simulink model "muxdemux"  (R2019b)
settings: Solver=VariableStepAuto  StartTime=0.0  StopTime=10.0  RelTol=1e-3
settings Model: Creator=Admin  LastModifiedBy=Admin

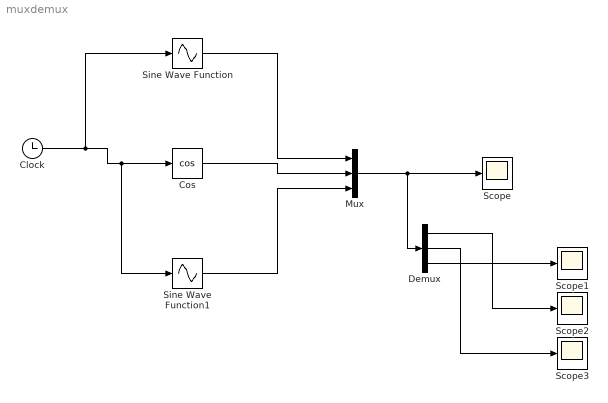
== system muxdemux ==
  Clock : Clock
  Cos : Trigonometry  Operator=cos
  Demux : Demux  Outputs=3
  Mux : Mux  Inputs=3
  Scope{,1..3} (4 alike) : Scope
  Sine Wave Function : Sin  TimeSource=Use external signal  SampleTime=0
  Sine Wave Function1 : Sin  TimeSource=Use external signal  Amplitude=2  SampleTime=0
  wires:
  Clock/1 -> Sine Wave Function/1, Sine Wave Function1/1, Cos/1
  Sine Wave Function/1 -> Mux/1
  Cos/1 -> Mux/2
  Sine Wave Function1/1 -> Mux/3
  Mux/1 -> Demux/1, Scope/1
  Demux/3 -> Scope1/1
  Demux/1 -> Scope2/1
  Demux/2 -> Scope3/1
